simulink model "g2_PI_kom_01"  (R2024a)
settings: Solver=ode1  StartTime=0.0  StopTime=7  FixedStep=Ts  RelTol=1e-3
PostLoadFcn:
  | GL_cbfcn('PostLoadFcn');
InitFcn:
  | GL_cbfcn('InitFcn');
StartFcn:
  | GL_cbfcn('StartFcn');
undefined symbols (not defined in the file or in its folder): burblks, DiscIntNeverNeededParam
libraries: bur_blks x1, cstblocks x1
(part 1 of 2)
PreSaveFcn:
  | GL_cbfcn('PreSaveFcn');
PostSaveFcn:
  | GL_cbfcn('PostSaveFcn');
CloseFcn:
  | GL_cbfcn('CloseFcn');
settings Model: GhostLab=GhostLab  GhostLab_ModelName=DCmot1  GhostLab_Version=2.0.4  CheckSum_Model=3683172000_965023117_984134679_3039741332  AS_Version=1.1.1  ExtModeTrigDuration=10000000  Creator=fldr  LastModifiedBy=rueegan5
settings DataIOCC: SaveFormat=Array  SaveOutput=off  SignalLogging=off  DSMLogging=off  SaveTime=off  ReturnWorkspaceOutputs=off
settings OptimizationCC: OptimizeBlockIOStorage=off  BufferReuse=off  GlobalBufferReuse=off  ExpressionFolding=off  EnableMemcpy=off  LocalBlockOutputs=off  InitFltsAndDblsToZero=on  LifeSpan=inf  OptimizeDataStoreBuffers=off  BusAssignmentInplaceUpdate=off
settings DebuggingCC: SaveWithDisabledLinksMsg=none  UnderspecifiedInitializationDetection=Classic  MergeDetectMultiDrivingBlocksExec=none  SolverPrmCheckMsg=warning  InheritedTsInSrcMsg=none  FcnCallInpInsideContextMsg=warning  FrameProcessingCompatibilityMsg=none  ModelReferenceSymbolNameMessage=none  StateNameClashWarn=warning  SFUnexpectedBacktrackingDiag=warning  SFNoUnconditionalDefaultTransitionDiag=warning
settings HardwareCC: ProdBitPerPointer=32  ProdBitPerSizeT=32  ProdBitPerPtrDiffT=32  ProdLargestAtomicFloat=None  ProdWordSize=32  ProdHWDeviceType=Intel->x86/Pentium
settings ModelReferenceCC: UpdateModelReferenceTargets=IfOutOfDate  ModelReferencePassRootInputsByReference=off  PropagateSignalLabelsOutOfModel=off
settings RTWCC: Description=B&R Automation Studio Target (GRT based)  SystemTargetFile=bur_grt.tlc  GenerateMakefile=off  TemplateMakefile=bur.tmf  RTWVerbose=off
settings RTWCC: CustomInitializer=|
  | udCheckSum0 = (0123456789U);
  | udCheckSum1 = (0123456789U);
  | udCheckSum2 = (0123456789U);
  | udCheckSum3 = (0123456789U);
  | udCurrentTime = &g2_PI_kom_01_M->Timing.t[0];
  | udclockTick0 = &g2_PI_kom_01_M->Timing.clockTick0;
  | udclockTickH0 = &g2_PI_kom_01_M->Timing.clockTickH0;
  | udParam = &g2_PI_kom_01_P;
  | udContinuousStates = &g2_PI_kom_01_X;
  | udDiscreteStates = &g2_PI_kom_01_DW;
settings CodeAppCC: MaxIdLength=255
settings STFCustomTargetCC: TargetLangStandard=C89/C90 (ANSI)  ParMdlRefBuildCompliant=on  UseToolchainInfoCompliant=off  SystemTargetFile=bur_grt.tlc
settings GRTTargetCC: TargetLangStandard=C89/C90 (ANSI)  CompOptLevelCompliant=off  ConcurrentExecutionCompliant=off  CombineOutputUpdateFcns=off  MatFileLogging=off  CPPClassGenCompliant=off  GRTInterface=on  UseToolchainInfoCompliant=off  ExtModeMexArgs='127.0.0.1'

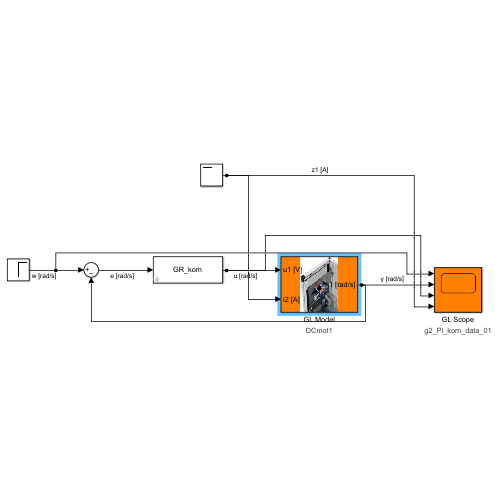
[thumbnail: Simulink's stored preview of the top-level diagram]
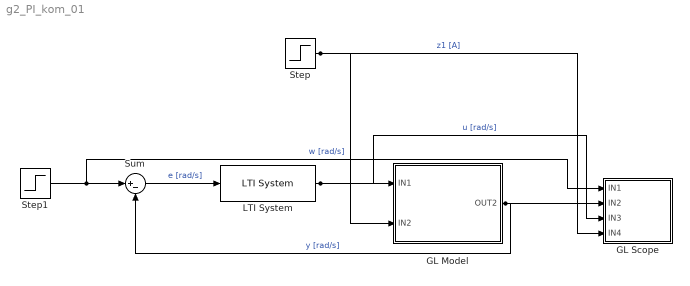
== system g2_PI_kom_01 ==
  GL Model : Subsystem  Tag=DCmot1  Description=GL_SetupModel;  mask(GhostLab Model){}
      settings: AttributesFormatString=%<Tag>  CopyFcn=GL_CopyFcn;  DeleteFcn=GL_cbfcn('Blk_DeleteFcn');  UndoDeleteFcn=GL_CopyFcn('BoW');  PreCopyFcn=GL_cbfcn('Blk_PreCopyFcn');  OpenFcn=GL_SetupModel;
      mask Display: image('DCmot1.png',[0.25,0,0.5,1]);color('black');port_label('input', 1, 'u1 [V]');port_label('input', 2, 'i2 [A]');port_label('output', 1, 'om1 [rad/s]');
  GL Scope : Subsystem  Tag=g2_PI_kom_data_01  Description=GL_cbfcn('openMask')  mask(GhostLab Scope){varname=g2_PI_kom_data_01, NumInputs=4, In1=1, In2=1, In3=1, In4=1, In5=1, In6=1, In7=1, In8=1, In9=1, In10=1}
      mask prompts: varname "Workspace Variable Name:"; NumInputs "Number of Input Ports:"; In1 "Input1:"; In2 "Input2:"; In3 "Input3:"; In4 "Input4:"; In5 "Input5:"; In6 "Input6:"; In7 "Input7:"; In8 "Input8:"; In9 "Input9:"; In10 "Input10:"
      mask help: View signals in GhostLab-App Scope-Tab and log data to workspace in structure with time format.
      mask init:
      | GL_cbfcn('updateScope');
      settings: AttributesFormatString=%<Tag>  CopyFcn=GL_cbfcn('copyGPA',gcb,'data');  DeleteFcn=GL_cbfcn('deleteScope');  UndoDeleteFcn=GL_cbfcn('updateScope');  OpenFcn=GL_cbfcn('openMask');
      mask Help: 1.0.2
      mask Callback varname: GL_cbfcn('set_var_name');
      mask TypeOptions NumInputs: 1 | 2 | 3 | 4 | 5 | 6 | 7 | 8 | 9
      mask Callback NumInputs: GL_cbfcn('updateScope');
      mask TypeOptions In1: 1 | 2 | 3
      mask Callback In1: %GL_cbfcn('updateScope');
      mask TypeOptions In2: 1 | 2 | 3
      mask Callback In2: %GL_cbfcn('updateScope');
      mask TypeOptions In3: 1 | 2 | 3
      mask Callback In3: %GL_cbfcn('updateScope');
      mask TypeOptions In4: 1 | 2 | 3
      mask Callback In4: %GL_cbfcn('updateScope');
      mask TypeOptions In5: 1 | 2 | 3
      mask Callback In5: %GL_cbfcn('updateScope');
      mask TypeOptions In6: 1 | 2 | 3
      mask Callback In6: %GL_cbfcn('updateScope');
      mask TypeOptions In7: 1 | 2 | 3
      mask Callback In7: %GL_cbfcn('updateScope');
      mask TypeOptions In8: 1 | 2 | 3
      mask Callback In8: %GL_cbfcn('updateScope');
      mask TypeOptions In9: 1 | 2 | 3
      mask Callback In9: %GL_cbfcn('updateScope');
      mask TypeOptions In10: 1 | 2 | 3
      mask Callback In10: %GL_cbfcn('updateScope');
      mask DialogControl Container3 Prompt: Log data to the following variable:
      mask DialogControl Container5 Prompt: Plot Signals in individual Axes:
      mask DialogControl Container4 Prompt: Signal Dimension for each Port
      mask Display: image(fullfile(fileparts(which('GhostLab')),'resources','icons','scope.png'));port_label('input', 1, '');
  LTI System : cstblocks/LTI System  sys=GR_kom  IC=[]  PadeOrder=0
  Step : Step  Time=4  After=-0.6  SampleTime=0
  Step1 : Step  After=15  SampleTime=0
  Sum : Sum  Inputs=|+-
  wires:
  Step/1 -> GL Scope/4(IN4), GL Model/2(IN2)  "z1 [A]"
  LTI System/1 -> GL Scope/3(IN3), GL Model/1(IN1)  "u [rad/s]"
  Sum/1 -> LTI System/1  "e [rad/s]"
  Step1/1 -> GL Scope/1(IN1), Sum/1  "w [rad/s]"
  GL Model/1(OUT2) -> GL Scope/2(IN2), Sum/2  "y [rad/s]"

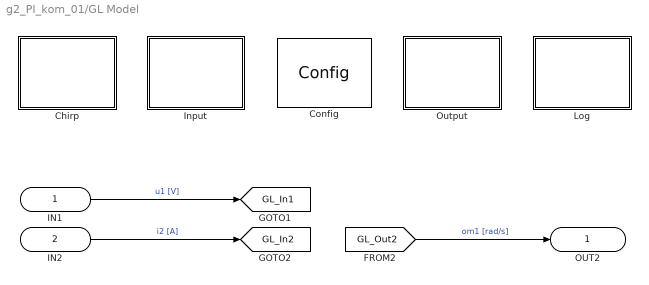
== system g2_PI_kom_01/GL Model ==
  IN1 : Inport
  IN2 : Inport  Port=2
  Chirp : Subsystem
  Config : bur_blks/Config  Tag=Coder: GRT C Target: Task  Description=burblks.classes.blks.BR_ConfigBlock.Do('open', gcb);  bur_configset_ert=C - Code Generation (Embedded Real Time Target based)  bur_configset_grt=C - Code Generation (Generic Real Time Target based)  bur_maskHandle=-1
      settings: AttributesFormatString=%<Tag>  SourceProductName=B&R Automation Studio Toolbox
  Input : Subsystem
  Log : Subsystem
  Output : Subsystem
  OUT2 : Outport
  tag scope: GL_In1=global, GL_In2=global
  wires:
  IN1/1 -> [GL_In1]  "u1 [V]"
  IN2/1 -> [GL_In2]  "i2 [A]"
  [GL_Out2] -> OUT2/1  "om1 [rad/s]"

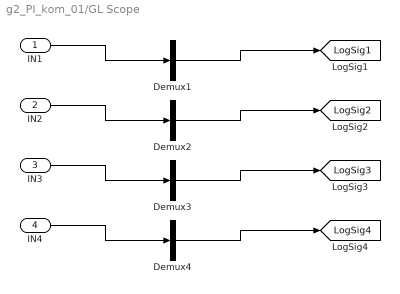
== system g2_PI_kom_01/GL Scope ==
  IN1 : Inport
  IN2 : Inport  Port=2
  IN3 : Inport  Port=3
  IN4 : Inport  Port=4
  Demux{1..4} (4 alike) : Demux  Outputs=1
  tag scope: LogSig1=global, LogSig2=global, LogSig3=global, LogSig4=global
  wires:
  IN1/1 -> Demux1/1
  Demux1/1 -> [LogSig1]
  IN2/1 -> Demux2/1
  Demux2/1 -> [LogSig2]
  IN3/1 -> Demux3/1
  Demux3/1 -> [LogSig3]
  IN4/1 -> Demux4/1
  Demux4/1 -> [LogSig4]

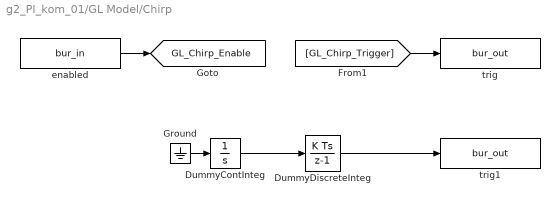
== system g2_PI_kom_01/GL Model/Chirp ==
  DummyContInteg : Integrator
  DummyDiscreteInteg : DiscreteIntegrator  SampleTime=-1  OutDataTypeStr=single  ICPrevOutput=DiscIntNeverNeededParam  ICPrevScaledInput=DiscIntNeverNeededParam
  Ground : Ground
  enabled : S-Function  Tag=GLOBAL BOOL bConnectionEstablished  Description=burblks.classes.blks.BR_InputBlock.Do('open', gcb)  LoadFcn=burblks.classes.blks.BR_InputBlock.Do( 'load', gcb)  InitFcn=burblks.classes.blks.BR_InputBlock.Do('init', gcb)  FunctionName=bur_in  Parameters=bur_scope, bur_data_type, bur_init_value, bur_init_value_bool, bur_array_index, bur_var_name, bur_AS_string  SFunctionDeploymentMode=off  EnableBusSupport=off  mask(B&&R - Input Block){bur_var_name=bConnectionEstablished, bur_var_description=, bur_scope=GLOBAL, bur_data_type=BOOL, bur_init_value=0, bur_init_value_bool=FALSE, bur_array_index=0, bur_old_var_name=, bur_var_memory=standard, bur_in_parameter=off, bur_AS_string=bConnectionEstablished : BOOL := 0; (**), bur_array_index_string=0}
      mask prompts: bur_var_name "Variable Name"; bur_var_description "Variable Description"; bur_scope "Variable Scope"; bur_data_type "Variable Data Type"; bur_init_value "Initial Value"; bur_init_value_bool "Initial Value"; bur_array_index "Array Dimension (0...Scalar)"; bur_old_var_name "Old Variable Name"; bur_var_memory "Memory"; bur_in_parameter "Parameter"; bur_array_index_string "Array Dimension Variable (0..Scalar)"
      mask help: Input interface for B&R Automation Studio process variable.
      settings: AttributesFormatString=%<Tag>  CopyFcn=burblks.classes.blks.BR_InputBlock.Do('copy', gcb)  DeleteFcn=burblks.classes.blks.BR_InputBlock.Do( 'delete', gcb)  ModelCloseFcn=burblks.classes.blks.BR_InputBlock.Do('close', gcb)  PreSaveFcn=burblks.classes.blks.BR_InputBlock.Do('preSave', gcb)  PostSaveFcn=burblks.classes.blks.BR_InputBlock.Do('postSave', gcb)  OpenFcn=burblks.classes.blks.BR_InputBlock.Do('open', gcb)
      mask Help: eval('burblks.classes.blks.BR_BlockHelp.Help(''InputBlock'')')
      mask TypeOptions bur_scope: GLOBAL | LOCAL
      mask TypeOptions bur_data_type: LREAL | REAL | SINT | USINT | INT | UINT | DINT | UDINT | BOOL | STRING
      mask TypeOptions bur_init_value_bool: FALSE | TRUE
      mask TypeOptions bur_var_memory: standard | retain
      mask Display: color('orange'); disp('B&R IN');
  trig : S-Function  Tag=GLOBAL BOOL bGPAtrigger  Description=burblks.classes.blks.BR_OutputBlock.Do('open', gcb)  LoadFcn=burblks.classes.blks.BR_OutputBlock.Do( 'load', gcb)  InitFcn=burblks.classes.blks.BR_OutputBlock.Do('init', gcb)  FunctionName=bur_out  Parameters=bur_scope, bur_data_type, bur_init_value, bur_init_value_bool, bur_array_index, bur_var_name, bur_AS_string  SFunctionDeploymentMode=off  EnableBusSupport=off  mask(B&&R - Output Block){bur_var_name=bGPAtrigger, bur_var_description=, bur_scope=GLOBAL, bur_data_type=BOOL, bur_init_value=0, bur_init_value_bool=FALSE, bur_array_index=0, bur_old_var_name=, bur_var_memory=standard, bur_AS_string=bGPAtrigger : BOOL := 0; (**), bur_array_index_string=0}
      mask prompts: bur_var_name "Variable Name"; bur_var_description "Variable Description"; bur_scope "Variable Scope"; bur_data_type "Variable Data Type"; bur_init_value "Initial Value"; bur_init_value_bool "Initial Value"; bur_array_index "Array Dimension (0...Scalar)"; bur_old_var_name "Old Variable Name"; bur_var_memory "Memory"; bur_array_index_string "Array Dimension Variable (0..Scalar)"
      mask help: Output interface for B&R Automation Studio process variable.
      settings: AttributesFormatString=%<Tag>  CopyFcn=burblks.classes.blks.BR_OutputBlock.Do('copy', gcb)  DeleteFcn=burblks.classes.blks.BR_OutputBlock.Do( 'delete', gcb)  ModelCloseFcn=burblks.classes.blks.BR_OutputBlock.Do('close', gcb)  PreSaveFcn=burblks.classes.blks.BR_OutputBlock.Do('preSave', gcb)  PostSaveFcn=burblks.classes.blks.BR_OutputBlock.Do('postSave', gcb)  OpenFcn=burblks.classes.blks.BR_OutputBlock.Do('open', gcb)
      mask Help: eval('burblks.classes.blks.BR_BlockHelp.Help(''OutputBlock'')')
      mask TypeOptions bur_scope: GLOBAL | LOCAL
      mask TypeOptions bur_data_type: LREAL | REAL | SINT | USINT | INT | UINT | DINT | UDINT | BOOL | STRING
      mask TypeOptions bur_init_value_bool: FALSE | TRUE
      mask TypeOptions bur_var_memory: standard | retain
      mask Display: color('orange'); disp('B&R OUT');
  trig1 : S-Function  Tag=GLOBAL REAL rDummy  Description=burblks.classes.blks.BR_OutputBlock.Do('open', gcb)  LoadFcn=burblks.classes.blks.BR_OutputBlock.Do( 'load', gcb)  InitFcn=burblks.classes.blks.BR_OutputBlock.Do('init', gcb)  FunctionName=bur_out  Parameters=bur_scope, bur_data_type, bur_init_value, bur_init_value_bool, bur_array_index, bur_var_name, bur_AS_string  SFunctionDeploymentMode=off  EnableBusSupport=off  mask(B&&R - Output Block){bur_var_name=rDummy, bur_var_description=, bur_scope=GLOBAL, bur_data_type=REAL, bur_init_value=0, bur_init_value_bool=FALSE, bur_array_index=0, bur_old_var_name=, bur_var_memory=standard, bur_AS_string=rDummy : REAL := 0; (**), bur_array_index_string=0}
      mask prompts: bur_var_name "Variable Name"; bur_var_description "Variable Description"; bur_scope "Variable Scope"; bur_data_type "Variable Data Type"; bur_init_value "Initial Value"; bur_init_value_bool "Initial Value"; bur_array_index "Array Dimension (0...Scalar)"; bur_old_var_name "Old Variable Name"; bur_var_memory "Memory"; bur_array_index_string "Array Dimension Variable (0..Scalar)"
      mask help: Output interface for B&R Automation Studio process variable.
      settings: AttributesFormatString=%<Tag>  CopyFcn=burblks.classes.blks.BR_OutputBlock.Do('copy', gcb)  DeleteFcn=burblks.classes.blks.BR_OutputBlock.Do( 'delete', gcb)  ModelCloseFcn=burblks.classes.blks.BR_OutputBlock.Do('close', gcb)  PreSaveFcn=burblks.classes.blks.BR_OutputBlock.Do('preSave', gcb)  PostSaveFcn=burblks.classes.blks.BR_OutputBlock.Do('postSave', gcb)  OpenFcn=burblks.classes.blks.BR_OutputBlock.Do('open', gcb)
      mask Help: eval('burblks.classes.blks.BR_BlockHelp.Help(''OutputBlock'')')
      mask TypeOptions bur_scope: GLOBAL | LOCAL
      mask TypeOptions bur_data_type: LREAL | REAL | SINT | USINT | INT | UINT | DINT | UDINT | BOOL | STRING
      mask TypeOptions bur_init_value_bool: FALSE | TRUE
      mask TypeOptions bur_var_memory: standard | retain
      mask Display: color('orange'); disp('B&R OUT');
  tag scope: GL_Chirp_Enable=global
  wires:
  [GL_Chirp_Trigger] -> trig/1
  enabled/1 -> [GL_Chirp_Enable]
  DummyContInteg/1 -> DummyDiscreteInteg/1
  Ground/1 -> DummyContInteg/1
  DummyDiscreteInteg/1 -> trig1/1

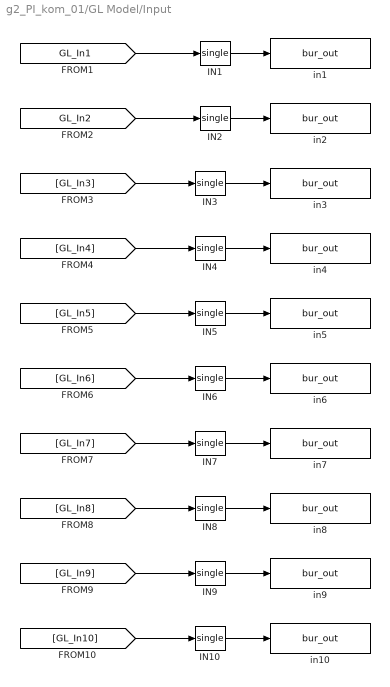
== system g2_PI_kom_01/GL Model/Input ==
  IN{1..10} (10 alike) : DataTypeConversion  OutDataTypeStr=single  SaturateOnIntegerOverflow=off  RndMeth=Floor
  in1 : S-Function  Tag=GLOBAL REAL rSimInput1  Description=burblks.classes.blks.BR_OutputBlock.Do('open', gcb)  LoadFcn=burblks.classes.blks.BR_OutputBlock.Do( 'load', gcb)  InitFcn=burblks.classes.blks.BR_OutputBlock.Do('init', gcb)  FunctionName=bur_out  Parameters=bur_scope, bur_data_type, bur_init_value, bur_init_value_bool, bur_array_index, bur_var_name, bur_AS_string  SFunctionDeploymentMode=off  EnableBusSupport=off  mask(B&&R - Output Block){bur_var_name=rSimInput1, bur_var_description=, bur_scope=GLOBAL, bur_data_type=REAL, bur_init_value=0, bur_init_value_bool=FALSE, bur_array_index=0, bur_old_var_name=, bur_var_memory=standard, bur_AS_string=rSimInput1 : REAL := 0; (**), bur_array_index_string=0}
      mask prompts: bur_var_name "Variable Name"; bur_var_description "Variable Description"; bur_scope "Variable Scope"; bur_data_type "Variable Data Type"; bur_init_value "Initial Value"; bur_init_value_bool "Initial Value"; bur_array_index "Array Dimension (0...Scalar)"; bur_old_var_name "Old Variable Name"; bur_var_memory "Memory"; bur_array_index_string "Array Dimension Variable (0..Scalar)"
      mask help: Output interface for B&R Automation Studio process variable.
      settings: AttributesFormatString=%<Tag>  CopyFcn=burblks.classes.blks.BR_OutputBlock.Do('copy', gcb)  DeleteFcn=burblks.classes.blks.BR_OutputBlock.Do( 'delete', gcb)  ModelCloseFcn=burblks.classes.blks.BR_OutputBlock.Do('close', gcb)  PreSaveFcn=burblks.classes.blks.BR_OutputBlock.Do('preSave', gcb)  PostSaveFcn=burblks.classes.blks.BR_OutputBlock.Do('postSave', gcb)  OpenFcn=burblks.classes.blks.BR_OutputBlock.Do('open', gcb)
      mask Help: eval('burblks.classes.blks.BR_BlockHelp.Help(''OutputBlock'')')
      mask TypeOptions bur_scope: GLOBAL | LOCAL
      mask TypeOptions bur_data_type: LREAL | REAL | SINT | USINT | INT | UINT | DINT | UDINT | BOOL | STRING
      mask TypeOptions bur_init_value_bool: FALSE | TRUE
      mask TypeOptions bur_var_memory: standard | retain
      mask Display: color('orange'); disp('B&R OUT');
  in10 : S-Function  Tag=GLOBAL REAL rSimInput10  Description=burblks.classes.blks.BR_OutputBlock.Do('open', gcb)  LoadFcn=burblks.classes.blks.BR_OutputBlock.Do( 'load', gcb)  InitFcn=burblks.classes.blks.BR_OutputBlock.Do('init', gcb)  FunctionName=bur_out  Parameters=bur_scope, bur_data_type, bur_init_value, bur_init_value_bool, bur_array_index, bur_var_name, bur_AS_string  SFunctionDeploymentMode=off  EnableBusSupport=off  mask(B&&R - Output Block){bur_var_name=rSimInput10, bur_var_description=, bur_scope=GLOBAL, bur_data_type=REAL, bur_init_value=0, bur_init_value_bool=FALSE, bur_array_index=0, bur_old_var_name=, bur_var_memory=standard, bur_AS_string=rSimInput10 : REAL := 0; (**), bur_array_index_string=0}
      mask prompts: bur_var_name "Variable Name"; bur_var_description "Variable Description"; bur_scope "Variable Scope"; bur_data_type "Variable Data Type"; bur_init_value "Initial Value"; bur_init_value_bool "Initial Value"; bur_array_index "Array Dimension (0...Scalar)"; bur_old_var_name "Old Variable Name"; bur_var_memory "Memory"; bur_array_index_string "Array Dimension Variable (0..Scalar)"
      mask help: Output interface for B&R Automation Studio process variable.
      settings: AttributesFormatString=%<Tag>  CopyFcn=burblks.classes.blks.BR_OutputBlock.Do('copy', gcb)  DeleteFcn=burblks.classes.blks.BR_OutputBlock.Do( 'delete', gcb)  ModelCloseFcn=burblks.classes.blks.BR_OutputBlock.Do('close', gcb)  PreSaveFcn=burblks.classes.blks.BR_OutputBlock.Do('preSave', gcb)  PostSaveFcn=burblks.classes.blks.BR_OutputBlock.Do('postSave', gcb)  OpenFcn=burblks.classes.blks.BR_OutputBlock.Do('open', gcb)
      mask Help: eval('burblks.classes.blks.BR_BlockHelp.Help(''OutputBlock'')')
      mask TypeOptions bur_scope: GLOBAL | LOCAL
      mask TypeOptions bur_data_type: LREAL | REAL | SINT | USINT | INT | UINT | DINT | UDINT | BOOL | STRING
      mask TypeOptions bur_init_value_bool: FALSE | TRUE
      mask TypeOptions bur_var_memory: standard | retain
      mask Display: color('orange'); disp('B&R OUT');
  in2 : S-Function  Tag=GLOBAL REAL rSimInput2  Description=burblks.classes.blks.BR_OutputBlock.Do('open', gcb)  LoadFcn=burblks.classes.blks.BR_OutputBlock.Do( 'load', gcb)  InitFcn=burblks.classes.blks.BR_OutputBlock.Do('init', gcb)  FunctionName=bur_out  Parameters=bur_scope, bur_data_type, bur_init_value, bur_init_value_bool, bur_array_index, bur_var_name, bur_AS_string  SFunctionDeploymentMode=off  EnableBusSupport=off  mask(B&&R - Output Block){bur_var_name=rSimInput2, bur_var_description=, bur_scope=GLOBAL, bur_data_type=REAL, bur_init_value=0, bur_init_value_bool=FALSE, bur_array_index=0, bur_old_var_name=, bur_var_memory=standard, bur_AS_string=rSimInput2 : REAL := 0; (**), bur_array_index_string=0}
      mask prompts: bur_var_name "Variable Name"; bur_var_description "Variable Description"; bur_scope "Variable Scope"; bur_data_type "Variable Data Type"; bur_init_value "Initial Value"; bur_init_value_bool "Initial Value"; bur_array_index "Array Dimension (0...Scalar)"; bur_old_var_name "Old Variable Name"; bur_var_memory "Memory"; bur_array_index_string "Array Dimension Variable (0..Scalar)"
      mask help: Output interface for B&R Automation Studio process variable.
      settings: AttributesFormatString=%<Tag>  CopyFcn=burblks.classes.blks.BR_OutputBlock.Do('copy', gcb)  DeleteFcn=burblks.classes.blks.BR_OutputBlock.Do( 'delete', gcb)  ModelCloseFcn=burblks.classes.blks.BR_OutputBlock.Do('close', gcb)  PreSaveFcn=burblks.classes.blks.BR_OutputBlock.Do('preSave', gcb)  PostSaveFcn=burblks.classes.blks.BR_OutputBlock.Do('postSave', gcb)  OpenFcn=burblks.classes.blks.BR_OutputBlock.Do('open', gcb)
      mask Help: eval('burblks.classes.blks.BR_BlockHelp.Help(''OutputBlock'')')
      mask TypeOptions bur_scope: GLOBAL | LOCAL
      mask TypeOptions bur_data_type: LREAL | REAL | SINT | USINT | INT | UINT | DINT | UDINT | BOOL | STRING
      mask TypeOptions bur_init_value_bool: FALSE | TRUE
      mask TypeOptions bur_var_memory: standard | retain
      mask Display: color('orange'); disp('B&R OUT');
  in3 : S-Function  Tag=GLOBAL REAL rSimInput3  Description=burblks.classes.blks.BR_OutputBlock.Do('open', gcb)  LoadFcn=burblks.classes.blks.BR_OutputBlock.Do( 'load', gcb)  InitFcn=burblks.classes.blks.BR_OutputBlock.Do('init', gcb)  FunctionName=bur_out  Parameters=bur_scope, bur_data_type, bur_init_value, bur_init_value_bool, bur_array_index, bur_var_name, bur_AS_string  SFunctionDeploymentMode=off  EnableBusSupport=off  mask(B&&R - Output Block){bur_var_name=rSimInput3, bur_var_description=, bur_scope=GLOBAL, bur_data_type=REAL, bur_init_value=0, bur_init_value_bool=FALSE, bur_array_index=0, bur_old_var_name=, bur_var_memory=standard, bur_AS_string=rSimInput3 : REAL := 0; (**), bur_array_index_string=0}
      mask prompts: bur_var_name "Variable Name"; bur_var_description "Variable Description"; bur_scope "Variable Scope"; bur_data_type "Variable Data Type"; bur_init_value "Initial Value"; bur_init_value_bool "Initial Value"; bur_array_index "Array Dimension (0...Scalar)"; bur_old_var_name "Old Variable Name"; bur_var_memory "Memory"; bur_array_index_string "Array Dimension Variable (0..Scalar)"
      mask help: Output interface for B&R Automation Studio process variable.
      settings: AttributesFormatString=%<Tag>  CopyFcn=burblks.classes.blks.BR_OutputBlock.Do('copy', gcb)  DeleteFcn=burblks.classes.blks.BR_OutputBlock.Do( 'delete', gcb)  ModelCloseFcn=burblks.classes.blks.BR_OutputBlock.Do('close', gcb)  PreSaveFcn=burblks.classes.blks.BR_OutputBlock.Do('preSave', gcb)  PostSaveFcn=burblks.classes.blks.BR_OutputBlock.Do('postSave', gcb)  OpenFcn=burblks.classes.blks.BR_OutputBlock.Do('open', gcb)
      mask Help: eval('burblks.classes.blks.BR_BlockHelp.Help(''OutputBlock'')')
      mask TypeOptions bur_scope: GLOBAL | LOCAL
      mask TypeOptions bur_data_type: LREAL | REAL | SINT | USINT | INT | UINT | DINT | UDINT | BOOL | STRING
      mask TypeOptions bur_init_value_bool: FALSE | TRUE
      mask TypeOptions bur_var_memory: standard | retain
      mask Display: color('orange'); disp('B&R OUT');
  in4 : S-Function  Tag=GLOBAL REAL rSimInput4  Description=burblks.classes.blks.BR_OutputBlock.Do('open', gcb)  LoadFcn=burblks.classes.blks.BR_OutputBlock.Do( 'load', gcb)  InitFcn=burblks.classes.blks.BR_OutputBlock.Do('init', gcb)  FunctionName=bur_out  Parameters=bur_scope, bur_data_type, bur_init_value, bur_init_value_bool, bur_array_index, bur_var_name, bur_AS_string  SFunctionDeploymentMode=off  EnableBusSupport=off  mask(B&&R - Output Block){bur_var_name=rSimInput4, bur_var_description=, bur_scope=GLOBAL, bur_data_type=REAL, bur_init_value=0, bur_init_value_bool=FALSE, bur_array_index=0, bur_old_var_name=, bur_var_memory=standard, bur_AS_string=rSimInput4 : REAL := 0; (**), bur_array_index_string=0}
      mask prompts: bur_var_name "Variable Name"; bur_var_description "Variable Description"; bur_scope "Variable Scope"; bur_data_type "Variable Data Type"; bur_init_value "Initial Value"; bur_init_value_bool "Initial Value"; bur_array_index "Array Dimension (0...Scalar)"; bur_old_var_name "Old Variable Name"; bur_var_memory "Memory"; bur_array_index_string "Array Dimension Variable (0..Scalar)"
      mask help: Output interface for B&R Automation Studio process variable.
      settings: AttributesFormatString=%<Tag>  CopyFcn=burblks.classes.blks.BR_OutputBlock.Do('copy', gcb)  DeleteFcn=burblks.classes.blks.BR_OutputBlock.Do( 'delete', gcb)  ModelCloseFcn=burblks.classes.blks.BR_OutputBlock.Do('close', gcb)  PreSaveFcn=burblks.classes.blks.BR_OutputBlock.Do('preSave', gcb)  PostSaveFcn=burblks.classes.blks.BR_OutputBlock.Do('postSave', gcb)  OpenFcn=burblks.classes.blks.BR_OutputBlock.Do('open', gcb)
      mask Help: eval('burblks.classes.blks.BR_BlockHelp.Help(''OutputBlock'')')
      mask TypeOptions bur_scope: GLOBAL | LOCAL
      mask TypeOptions bur_data_type: LREAL | REAL | SINT | USINT | INT | UINT | DINT | UDINT | BOOL | STRING
      mask TypeOptions bur_init_value_bool: FALSE | TRUE
      mask TypeOptions bur_var_memory: standard | retain
      mask Display: color('orange'); disp('B&R OUT');
  in5 : S-Function  Tag=GLOBAL REAL rSimInput5  Description=burblks.classes.blks.BR_OutputBlock.Do('open', gcb)  LoadFcn=burblks.classes.blks.BR_OutputBlock.Do( 'load', gcb)  InitFcn=burblks.classes.blks.BR_OutputBlock.Do('init', gcb)  FunctionName=bur_out  Parameters=bur_scope, bur_data_type, bur_init_value, bur_init_value_bool, bur_array_index, bur_var_name, bur_AS_string  SFunctionDeploymentMode=off  EnableBusSupport=off  mask(B&&R - Output Block){bur_var_name=rSimInput5, bur_var_description=, bur_scope=GLOBAL, bur_data_type=REAL, bur_init_value=0, bur_init_value_bool=FALSE, bur_array_index=0, bur_old_var_name=, bur_var_memory=standard, bur_AS_string=rSimInput5 : REAL := 0; (**), bur_array_index_string=0}
      mask prompts: bur_var_name "Variable Name"; bur_var_description "Variable Description"; bur_scope "Variable Scope"; bur_data_type "Variable Data Type"; bur_init_value "Initial Value"; bur_init_value_bool "Initial Value"; bur_array_index "Array Dimension (0...Scalar)"; bur_old_var_name "Old Variable Name"; bur_var_memory "Memory"; bur_array_index_string "Array Dimension Variable (0..Scalar)"
      mask help: Output interface for B&R Automation Studio process variable.
      settings: AttributesFormatString=%<Tag>  CopyFcn=burblks.classes.blks.BR_OutputBlock.Do('copy', gcb)  DeleteFcn=burblks.classes.blks.BR_OutputBlock.Do( 'delete', gcb)  ModelCloseFcn=burblks.classes.blks.BR_OutputBlock.Do('close', gcb)  PreSaveFcn=burblks.classes.blks.BR_OutputBlock.Do('preSave', gcb)  PostSaveFcn=burblks.classes.blks.BR_OutputBlock.Do('postSave', gcb)  OpenFcn=burblks.classes.blks.BR_OutputBlock.Do('open', gcb)
      mask Help: eval('burblks.classes.blks.BR_BlockHelp.Help(''OutputBlock'')')
      mask TypeOptions bur_scope: GLOBAL | LOCAL
      mask TypeOptions bur_data_type: LREAL | REAL | SINT | USINT | INT | UINT | DINT | UDINT | BOOL | STRING
      mask TypeOptions bur_init_value_bool: FALSE | TRUE
      mask TypeOptions bur_var_memory: standard | retain
      mask Display: color('orange'); disp('B&R OUT');
  in6 : S-Function  Tag=GLOBAL REAL rSimInput6  Description=burblks.classes.blks.BR_OutputBlock.Do('open', gcb)  LoadFcn=burblks.classes.blks.BR_OutputBlock.Do( 'load', gcb)  InitFcn=burblks.classes.blks.BR_OutputBlock.Do('init', gcb)  FunctionName=bur_out  Parameters=bur_scope, bur_data_type, bur_init_value, bur_init_value_bool, bur_array_index, bur_var_name, bur_AS_string  SFunctionDeploymentMode=off  EnableBusSupport=off  mask(B&&R - Output Block){bur_var_name=rSimInput6, bur_var_description=, bur_scope=GLOBAL, bur_data_type=REAL, bur_init_value=0, bur_init_value_bool=FALSE, bur_array_index=0, bur_old_var_name=, bur_var_memory=standard, bur_AS_string=rSimInput6 : REAL := 0; (**), bur_array_index_string=0}
      mask prompts: bur_var_name "Variable Name"; bur_var_description "Variable Description"; bur_scope "Variable Scope"; bur_data_type "Variable Data Type"; bur_init_value "Initial Value"; bur_init_value_bool "Initial Value"; bur_array_index "Array Dimension (0...Scalar)"; bur_old_var_name "Old Variable Name"; bur_var_memory "Memory"; bur_array_index_string "Array Dimension Variable (0..Scalar)"
      mask help: Output interface for B&R Automation Studio process variable.
      settings: AttributesFormatString=%<Tag>  CopyFcn=burblks.classes.blks.BR_OutputBlock.Do('copy', gcb)  DeleteFcn=burblks.classes.blks.BR_OutputBlock.Do( 'delete', gcb)  ModelCloseFcn=burblks.classes.blks.BR_OutputBlock.Do('close', gcb)  PreSaveFcn=burblks.classes.blks.BR_OutputBlock.Do('preSave', gcb)  PostSaveFcn=burblks.classes.blks.BR_OutputBlock.Do('postSave', gcb)  OpenFcn=burblks.classes.blks.BR_OutputBlock.Do('open', gcb)
      mask Help: eval('burblks.classes.blks.BR_BlockHelp.Help(''OutputBlock'')')
      mask TypeOptions bur_scope: GLOBAL | LOCAL
      mask TypeOptions bur_data_type: LREAL | REAL | SINT | USINT | INT | UINT | DINT | UDINT | BOOL | STRING
      mask TypeOptions bur_init_value_bool: FALSE | TRUE
      mask TypeOptions bur_var_memory: standard | retain
      mask Display: color('orange'); disp('B&R OUT');
  in7 : S-Function  Tag=GLOBAL REAL rSimInput7  Description=burblks.classes.blks.BR_OutputBlock.Do('open', gcb)  LoadFcn=burblks.classes.blks.BR_OutputBlock.Do( 'load', gcb)  InitFcn=burblks.classes.blks.BR_OutputBlock.Do('init', gcb)  FunctionName=bur_out  Parameters=bur_scope, bur_data_type, bur_init_value, bur_init_value_bool, bur_array_index, bur_var_name, bur_AS_string  SFunctionDeploymentMode=off  EnableBusSupport=off  mask(B&&R - Output Block){bur_var_name=rSimInput7, bur_var_description=, bur_scope=GLOBAL, bur_data_type=REAL, bur_init_value=0, bur_init_value_bool=FALSE, bur_array_index=0, bur_old_var_name=, bur_var_memory=standard, bur_AS_string=rSimInput7 : REAL := 0; (**), bur_array_index_string=0}
      mask prompts: bur_var_name "Variable Name"; bur_var_description "Variable Description"; bur_scope "Variable Scope"; bur_data_type "Variable Data Type"; bur_init_value "Initial Value"; bur_init_value_bool "Initial Value"; bur_array_index "Array Dimension (0...Scalar)"; bur_old_var_name "Old Variable Name"; bur_var_memory "Memory"; bur_array_index_string "Array Dimension Variable (0..Scalar)"
      mask help: Output interface for B&R Automation Studio process variable.
      settings: AttributesFormatString=%<Tag>  CopyFcn=burblks.classes.blks.BR_OutputBlock.Do('copy', gcb)  DeleteFcn=burblks.classes.blks.BR_OutputBlock.Do( 'delete', gcb)  ModelCloseFcn=burblks.classes.blks.BR_OutputBlock.Do('close', gcb)  PreSaveFcn=burblks.classes.blks.BR_OutputBlock.Do('preSave', gcb)  PostSaveFcn=burblks.classes.blks.BR_OutputBlock.Do('postSave', gcb)  OpenFcn=burblks.classes.blks.BR_OutputBlock.Do('open', gcb)
      mask Help: eval('burblks.classes.blks.BR_BlockHelp.Help(''OutputBlock'')')
      mask TypeOptions bur_scope: GLOBAL | LOCAL
      mask TypeOptions bur_data_type: LREAL | REAL | SINT | USINT | INT | UINT | DINT | UDINT | BOOL | STRING
      mask TypeOptions bur_init_value_bool: FALSE | TRUE
      mask TypeOptions bur_var_memory: standard | retain
      mask Display: color('orange'); disp('B&R OUT');
  in8 : S-Function  Tag=GLOBAL REAL rSimInput8  Description=burblks.classes.blks.BR_OutputBlock.Do('open', gcb)  LoadFcn=burblks.classes.blks.BR_OutputBlock.Do( 'load', gcb)  InitFcn=burblks.classes.blks.BR_OutputBlock.Do('init', gcb)  FunctionName=bur_out  Parameters=bur_scope, bur_data_type, bur_init_value, bur_init_value_bool, bur_array_index, bur_var_name, bur_AS_string  SFunctionDeploymentMode=off  EnableBusSupport=off  mask(B&&R - Output Block){bur_var_name=rSimInput8, bur_var_description=, bur_scope=GLOBAL, bur_data_type=REAL, bur_init_value=0, bur_init_value_bool=FALSE, bur_array_index=0, bur_old_var_name=, bur_var_memory=standard, bur_AS_string=rSimInput8 : REAL := 0; (**), bur_array_index_string=0}
      mask prompts: bur_var_name "Variable Name"; bur_var_description "Variable Description"; bur_scope "Variable Scope"; bur_data_type "Variable Data Type"; bur_init_value "Initial Value"; bur_init_value_bool "Initial Value"; bur_array_index "Array Dimension (0...Scalar)"; bur_old_var_name "Old Variable Name"; bur_var_memory "Memory"; bur_array_index_string "Array Dimension Variable (0..Scalar)"
      mask help: Output interface for B&R Automation Studio process variable.
      settings: AttributesFormatString=%<Tag>  CopyFcn=burblks.classes.blks.BR_OutputBlock.Do('copy', gcb)  DeleteFcn=burblks.classes.blks.BR_OutputBlock.Do( 'delete', gcb)  ModelCloseFcn=burblks.classes.blks.BR_OutputBlock.Do('close', gcb)  PreSaveFcn=burblks.classes.blks.BR_OutputBlock.Do('preSave', gcb)  PostSaveFcn=burblks.classes.blks.BR_OutputBlock.Do('postSave', gcb)  OpenFcn=burblks.classes.blks.BR_OutputBlock.Do('open', gcb)
      mask Help: eval('burblks.classes.blks.BR_BlockHelp.Help(''OutputBlock'')')
      mask TypeOptions bur_scope: GLOBAL | LOCAL
      mask TypeOptions bur_data_type: LREAL | REAL | SINT | USINT | INT | UINT | DINT | UDINT | BOOL | STRING
      mask TypeOptions bur_init_value_bool: FALSE | TRUE
      mask TypeOptions bur_var_memory: standard | retain
      mask Display: color('orange'); disp('B&R OUT');
  in9 : S-Function  Tag=GLOBAL REAL rSimInput9  Description=burblks.classes.blks.BR_OutputBlock.Do('open', gcb)  LoadFcn=burblks.classes.blks.BR_OutputBlock.Do( 'load', gcb)  InitFcn=burblks.classes.blks.BR_OutputBlock.Do('init', gcb)  FunctionName=bur_out  Parameters=bur_scope, bur_data_type, bur_init_value, bur_init_value_bool, bur_array_index, bur_var_name, bur_AS_string  SFunctionDeploymentMode=off  EnableBusSupport=off  mask(B&&R - Output Block){bur_var_name=rSimInput9, bur_var_description=, bur_scope=GLOBAL, bur_data_type=REAL, bur_init_value=0, bur_init_value_bool=FALSE, bur_array_index=0, bur_old_var_name=, bur_var_memory=standard, bur_AS_string=rSimInput9 : REAL := 0; (**), bur_array_index_string=0}
      mask prompts: bur_var_name "Variable Name"; bur_var_description "Variable Description"; bur_scope "Variable Scope"; bur_data_type "Variable Data Type"; bur_init_value "Initial Value"; bur_init_value_bool "Initial Value"; bur_array_index "Array Dimension (0...Scalar)"; bur_old_var_name "Old Variable Name"; bur_var_memory "Memory"; bur_array_index_string "Array Dimension Variable (0..Scalar)"
      mask help: Output interface for B&R Automation Studio process variable.
      settings: AttributesFormatString=%<Tag>  CopyFcn=burblks.classes.blks.BR_OutputBlock.Do('copy', gcb)  DeleteFcn=burblks.classes.blks.BR_OutputBlock.Do( 'delete', gcb)  ModelCloseFcn=burblks.classes.blks.BR_OutputBlock.Do('close', gcb)  PreSaveFcn=burblks.classes.blks.BR_OutputBlock.Do('preSave', gcb)  PostSaveFcn=burblks.classes.blks.BR_OutputBlock.Do('postSave', gcb)  OpenFcn=burblks.classes.blks.BR_OutputBlock.Do('open', gcb)
      mask Help: eval('burblks.classes.blks.BR_BlockHelp.Help(''OutputBlock'')')
      mask TypeOptions bur_scope: GLOBAL | LOCAL
      mask TypeOptions bur_data_type: LREAL | REAL | SINT | USINT | INT | UINT | DINT | UDINT | BOOL | STRING
      mask TypeOptions bur_init_value_bool: FALSE | TRUE
      mask TypeOptions bur_var_memory: standard | retain
      mask Display: color('orange'); disp('B&R OUT');
  wires:
  IN5/1 -> in5/1
  IN8/1 -> in8/1
  [GL_In8] -> IN8/1
  IN9/1 -> in9/1
  [GL_In9] -> IN9/1
  IN6/1 -> in6/1
  IN3/1 -> in3/1
  [GL_In5] -> IN5/1
  [GL_In3] -> IN3/1
  [GL_In1] -> IN1/1
  [GL_In6] -> IN6/1
  IN2/1 -> in2/1
  [GL_In4] -> IN4/1
  IN10/1 -> in10/1
  [GL_In7] -> IN7/1
  [GL_In10] -> IN10/1
  IN1/1 -> in1/1
  IN4/1 -> in4/1
  IN7/1 -> in7/1
  [GL_In2] -> IN2/1
